simulink model "TeamA_PAsqualo1"  (R2020a)
settings: Solver=VariableStepAuto  StartTime=0.0  StopTime=stop_time  FixedStep=0.05  RelTol=1e-3
InitFcn:
  | main_init
values from neighbouring files (symbols this model uses):
  a1 = rho * D^4 * alpha1    (= 0.000388302366464)    [data_current.m]    (also in main_init.m)
  a2 = -rho * D^3 * alpha2 * (1 - omega)    (= 0.0037030698432)    [data_current.m]    (also in main_init.m)
  ag = [Ax Ay Az]'    [init_modello.m]
  alpha1 = 0.0113    [data_current.m]    (also in main_init.m)
  alpha2 = -0.0091    [data_current.m]    (also in main_init.m)
  areaOfInterestCorner = [42.317744;10.915136; 0]    [init_controllo.m]    (also in missionA.m = [42.317744)
  bg = [Bx By Bz]'    [init_modello.m]
  cd_pitch = 0.7    [init_modello.m]
  cd_roll = 0.04    [init_modello.m]
  cd_x = 0.4    [init_modello.m]
  cd_y = 1    [init_modello.m]
  cd_yaw = 0.7    [init_modello.m]
  cd_z = 1    [init_modello.m]
  cg = [Cx Cy Cz]'    [init_modello.m]
  D = 0.076    [data_current.m]    (also in main_init.m)
  dead_zone_limit = 31.5    [data_current.m]    (also in main_init.m)
  dg = [Dx Dy Dz]'    [init_modello.m]
  eg = [Ex Ey Ez]'    [init_modello.m]
  fg = [Fx Fy Fz]'    [init_modello.m]
  g = 9.81    [init_modello.m]
  galleggiamento = 66.5386    [init_controllo.m]
  gg = [Gx Gy Gz]'    [init_modello.m]
  H0 = 0    [init_modello.m]
  init_position = [pointP(1),pointP(2),0.15,0,0,deg2rad(angle)]'    [appunti.m]    (also in init_modello.m = [pointP(1),pointP(2),0.15,0,0,deg2rad(alpha)]')
  init_velocity = [0 0 0 0 0 0]'    [init_modello.m]
  initial_state_cov = blkdiag(diag(cov_gps(1,1:2)), cov_depth*eye(n_state_filter-2))    [init_navigazione.m]
  Ixx = 0.93304097392    [init_modello.m]
  Ixy = 0    [init_modello.m]
  Ixz = 0    [init_modello.m]
  Iyy = 25.58745481378    (= 25.5874548138)    [init_modello.m]
  Iyz = 0    [init_modello.m]
  Izz = 25.58745481378    (= 25.5874548138)    [init_modello.m]
  K_i_heave_div = 20    [init_controllo.m]
  K_i_heave_pos = 1    [init_controllo.m]
  K_i_heave_surf = 20    [init_controllo.m]
  K_i_heave_trans = 5    [init_controllo.m]
  K_i_heave_turn = 5    [init_controllo.m]
  K_i_pitch_div = 0    [init_controllo.m]
  K_i_pitch_pos = 0.1*0    (= 0)    [init_controllo.m]
  K_i_pitch_surf = 0    [init_controllo.m]
  K_i_pitch_trans = 0    [init_controllo.m]
  K_i_pitch_turn = 0    [init_controllo.m]
  K_i_roll_div = 0    [init_controllo.m]
  K_i_roll_pos = 0.1*0    (= 0)    [init_controllo.m]
  K_i_roll_surf = 1    [init_controllo.m]
  K_i_roll_trans = 0    [init_controllo.m]
  K_i_roll_turn = 0    [init_controllo.m]
  K_i_surge_div = 3    [init_controllo.m]
  K_i_surge_pos = 0.1679*30    (= 5.037)    [init_controllo.m]
  K_i_surge_surf = 3    [init_controllo.m]
  K_i_surge_trans = 0.1679*15    (= 2.5185)    [init_controllo.m]
  K_i_surge_turn = 0.1679*60    (= 10.074)    [init_controllo.m]
  K_i_sway_div = 6    [init_controllo.m]
  K_i_sway_pos = 5    [init_controllo.m]
  K_i_sway_surf = 3    [init_controllo.m]
  K_i_sway_trans = 2    [init_controllo.m]
  K_i_sway_turn = 50    [init_controllo.m]
  K_i_yaw_div = 0    [init_controllo.m]
  K_i_yaw_pos = 1    [init_controllo.m]
  K_i_yaw_surf = 0    [init_controllo.m]
  K_i_yaw_trans = 20    [init_controllo.m]
  K_i_yaw_turn = 3    [init_controllo.m]
  K_p_heave_div = 200    [init_controllo.m]
  K_p_heave_pos = 320    [init_controllo.m]
  K_p_heave_surf = 200    [init_controllo.m]
  K_p_heave_trans = 170    [init_controllo.m]
  K_p_heave_turn = 170    [init_controllo.m]
  K_p_phi_div = 0.15    [init_controllo.m]
  K_p_phi_pos = 1*0.1    (= 0.1)    [init_controllo.m]
  K_p_phi_surf = 0.15    [init_controllo.m]
  K_p_phi_trans = 0.1    [init_controllo.m]
  K_p_phi_turn = 0.1    [init_controllo.m]
  K_p_pitch_div = 50    [init_controllo.m]
  K_p_pitch_pos = 25    [init_controllo.m]
  K_p_pitch_surf = 50    [init_controllo.m]
  K_p_pitch_trans = 25    [init_controllo.m]
  K_p_pitch_turn = 25    [init_controllo.m]
  K_p_psi_div = 0.3    [init_controllo.m]
  K_p_psi_pos = 0.25    [init_controllo.m]
  K_p_psi_surf = 0.3    [init_controllo.m]
  K_p_psi_trans = 0.2    [init_controllo.m]
  K_p_roll_div = 10    [init_controllo.m]
  K_p_roll_pos = 0.1*40    (= 4)    [init_controllo.m]
  K_p_roll_surf = 10    [init_controllo.m]
  K_p_roll_trans = 0.1*40    (= 4)    [init_controllo.m]
  K_p_roll_turn = 4    [init_controllo.m]
  K_p_surge_div = 80    [init_controllo.m]
  K_p_surge_pos = 13.7782*2.5    (= 34.4455)    [init_controllo.m]
  K_p_surge_surf = 80    [init_controllo.m]
  K_p_surge_trans = 20    [init_controllo.m]
  K_p_surge_turn = 150    [init_controllo.m]
  K_p_sway_div = 100    [init_controllo.m]
  K_p_sway_pos = 90    [init_controllo.m]
  K_p_sway_surf = 80    [init_controllo.m]
  K_p_sway_trans = 80    [init_controllo.m]
  K_p_sway_turn = 200    [init_controllo.m]
  K_p_th_div = 0.3    [init_controllo.m]
  K_p_th_pos = 0.1    [init_controllo.m]
  K_p_th_surf = 0.3    [init_controllo.m]
  K_p_th_trans = 0.1    [init_controllo.m]
  K_p_th_turn = 0.1    [init_controllo.m]
  K_p_x_div = 0.12    [init_controllo.m]
  K_p_x_pos = 0.12    [init_controllo.m]
  K_p_x_surf = 0.12    [init_controllo.m]
  K_p_y_div = 0.6    [init_controllo.m]
  K_p_y_pos = 0.34    [init_controllo.m]
  K_p_y_surf = 0.1    [init_controllo.m]
  K_p_y_trans = 0.3    [init_controllo.m]
  K_p_y_turn = 0.3    [init_controllo.m]
  K_p_yaw_div = 70    [init_controllo.m]
  K_p_yaw_pos = 20    [init_controllo.m]
  K_p_yaw_surf = 70    [init_controllo.m]
  K_p_yaw_trans = 160    [init_controllo.m]
  K_p_yaw_turn = 60    [init_controllo.m]
  K_p_z_div = 0.35    [init_controllo.m]
  K_p_z_pos = 0.2    [init_controllo.m]
  K_p_z_surf = 0.35    [init_controllo.m]
  K_p_z_trans = 0.10    (= 0.1)    [init_controllo.m]
  K_p_z_turn = 0.1    [init_controllo.m]
  Kadd = 0    [init_modello.m]
  ... (+61 more)
undefined symbols (not defined in the file or in its folder): DiscIntNeverNeededParam, initial_state
libraries: simulink x4, vrlib x1
(part 4 of 6)

== matlab function TeamA_PAsqualo1/Navigazione/Predizione/predizione_propagate ==
  data: mean input size=[n_state_aug_filter 1]; mean_new output size=[n_state_filter, 1]; cov input size=[n_state_aug_filter n_state_aug_filter]; cov_new output size=[n_state_filter n_state_filter]; n_state_aug_filter parameter; ts_filter parameter; n_state_filter parameter
function [mean_new, cov_new] = propagate(mean, cov, n_state_aug_filter, ts_filter, n_state_filter)
 % PROPAGATE genera un numero n di sigma points, li propaga attraverso
 % state_update e da` come output la media e la covarianza dei nuovi sigma
 % points. 
 %
 % Input		
 % mean			vettore media dello stato nx1
 % cov			matrice covarianza dello stato nxn
 %
 % Output
 % mean_new		vettore media dello stato nx1
 % cov_new		matrice covarianza dello stato nxn

[sp, wm, wc] = sigmapoint_gen(mean, cov, n_state_aug_filter);

[mean_new, P] = sigmapoint_propagate(sp, wm, wc, ...
					n_state_aug_filter, ts_filter, n_state_filter);

% check simmetria
cov_new = (P + P')/2;

end

%--------------------------------------------------------------------------
%--------------------------------------------------------------------------
function state_new = state_update(state_aug, ts_filter)


pos = state_aug(1:3, 1);
ahrs = state_aug(4:6, 1); % roll pitch yaw
dvl = state_aug(7:9, 1);

% yaw, pitch, roll
Rbn = rotz(ahrs(3))' * roty(ahrs(2))' * rotx(ahrs(1))';

state_new = pos + ts_filter * Rbn * dvl;

end

function Rx = rotx(ang)

Rx = [	1 0 0; ...
		0 cos(ang) sin(ang); ...
		0 -sin(ang) cos(ang)];

end
function Ry = roty(ang)

Ry = [	cos(ang) 0 -sin(ang); ...
		0 1 0; ...
		sin(ang) 0 cos(ang)];

end
function Rz = rotz(ang)

Rz = [	cos(ang) sin(ang) 0; ...
		-sin(ang) cos(ang) 0; ...
		0	0 1];

end
		
%--------------------------------------------------------------------------
%--------------------------------------------------------------------------
function [sp, wm, wc] = sigmapoint_gen(mean, cov, n_state_filter)
% questa funzione genera i sigma point e i loro pesi
	

	n		= n_state_filter;	% Dimensione dello spazio in cui vengono generati
	nsp		= 2*n+1;			% numero di sigma points. in generale pari a (2n+1)
	P       = cov;				% matrice di covarianza
%	mean    = mean;				%
	
	% par da rivedere
	alpha	= 1;
	beta	= 2;
	k		= 0;
    
	%   
	lambda = alpha^2 * (n + k) -n;
	
	% generazione pesi per media
	wm = 1/(2*(n + lambda)) * ones(nsp, 1);
    wm(1) = lambda/(n + lambda);
	
	% generazione pesi per cov
	wc = 1/(2*(n + lambda)) * ones(nsp, 1);
	wc(1) = lambda/(n + lambda) + (1 - alpha^2 + beta);
	
	% generazione sigma points sp
	dist = zeros(n_state_filter,n_state_filter);
	sp = zeros(n_state_filter, nsp);
	
	[U, SIGMA, ~] = svd((n+lambda)* P);
	dist = U * sqrt(SIGMA);

	for i=1:nsp
		if i == 1
			sp(:,i) = mean;
		elseif i<=1+n
			sp(:,i) = mean+dist(:,i-1);
		elseif i>1+n && i<=nsp
			sp(:,i) = mean-dist(:,i-1-n);
		end
	end

end

%--------------------------------------------------------------------------
%--------------------------------------------------------------------------
function [mean_new, cov_new] = sigmapoint_propagate(sp, wm, wc, n_state_aug_filter, ts_filter, n_state_filter)
% questa funzione propaga i sigma point usando state_update
	
	
	nsp = n_state_aug_filter*2 + 1;
	sp_new = zeros(n_state_filter, nsp);
	for j = 1:nsp
		 sp_new(:,j) = state_update(sp(:,j), ts_filter);
	end

	% media
	mean_new = zeros(n_state_filter, 1);
	for j = 1:nsp
		mean_new = mean_new + wm(j)*sp_new(:,j);
	end

	% cov
	cov_new = zeros(n_state_filter, n_state_filter);  
	for j = 1:nsp
		 cov_new = cov_new + wc(j)*(sp_new(:,j) - mean_new)*(sp_new(:,j) - mean_new)';
	end

	
end

== matlab function TeamA_PAsqualo1/Navigazione/Predizione/smart_mux ==
  data: x_mean input size=[n_state_filter 1]; mean output size=[9 1]; x_cov input size=[n_state_filter n_state_filter]; u_mean input size=[n_input_filter 1]; u_cov input size=[n_input_filter n_input_filter]; cov output size=[n_state_aug_filter, n_state_aug_filter]; n_state_filter parameter; n_input_filter parameter
function [mean, cov] = smart_mux(x_mean, x_cov, u_mean, u_cov, n_state_filter, n_input_filter)

% init
mean = zeros(n_state_filter+n_input_filter, 1);
mean = [x_mean; u_mean];
    
cov = zeros(n_state_filter + n_input_filter);
cov = blkdiag(x_cov, u_cov);

end

== matlab function TeamA_PAsqualo1/Navigazione/Predizione Misure/propagazione misura NED1 ==
  data: x input; P input; y_virt output size=[5 1]; S_virt output; C output; n_state_filter parameter; n_meas_filter parameter; pos_transp parameter; p_usbl parameter; or input
function [y_virt, S_virt, C] = propagazione_misure(x, P, n_state_filter, n_meas_filter, pos_transp, p_usbl, or)
 % PROPAGATE_MISURE genera i sigma points, li propaga attraverso state2meas
 % e da` come output la media, la covarianza dei nuovi sigma points e la 
 % crosscovarianza stato-meas.
 %
 % Input		
 % mean			vettore media dello stato nx1
 % cov			matrice covarianza dello stato nxn
 %
 % Output
 % mean_new		vettore media dello misure mx1
 % cov_new		matrice covarianza dello delle misure mxm
 % C			matrice crosscovarianza nxm


[sp, wm, wc] = sigmapoint_gen(x, P, n_state_filter);

[~, y_virt, esse, C] = sigmapoint_propagate(sp, x, wm, wc, n_state_filter, ...
									n_meas_filter, pos_transp, p_usbl, or);

% check simmetria								
S_virt = (esse + esse')/2;


end

%--------------------------------------------------------------------------
%--------------------------------------------------------------------------
function meas = state2meas(state, n_meas_filter, pos_transp,  p_usbl, or)

meas = zeros(n_meas_filter,1);

Rbn = rotz(or(3))' * roty(or(2))' * rotx(or(1))';

% ned2usbl
pos_sensore_onboard = state(1:3,1) + Rbn*p_usbl;

vettore_auv_trasp =  +(pos_transp - pos_sensore_onboard) ;
range	= norm(vettore_auv_trasp,2);
bear	= atan2(vettore_auv_trasp(2),vettore_auv_trasp(1));

% depth
meas_depth = state(3);


meas = [state(1); state(2); bear; range; meas_depth];

end


function Rx = rotx(ang)

Rx = [	1 0 0; ...
		0 cos(ang) sin(ang); ...
		0 -sin(ang) cos(ang)];

end
function Ry = roty(ang)

Ry = [	cos(ang) 0 -sin(ang); ...
		0 1 0; ...
		sin(ang) 0 cos(ang)];

end
function Rz = rotz(ang)

Rz = [	cos(ang) sin(ang) 0; ...
		-sin(ang) cos(ang) 0; ...
		0	0 1];

end

%--------------------------------------------------------------------------
%--------------------------------------------------------------------------
function [sp, wm, wc] = sigmapoint_gen(mean, cov, n_state_filter)
% questa funzione genera i sigma point e i loro pesi


	n		= n_state_filter;	% Dimensione dello spazio in cui vengono generati
	nsp		= 2*n+1;			% numero di sigma points. in generale pari a (2n+1)
	P       = cov;				% matrice di covarianza
%	mean    = mean;				%
	
	% par da rivedere
	alpha	= 1;
	beta	= 2;
	k		= 0;
    
	%   
	lambda = alpha^2 * (n + k) -n;
	
	% generazione pesi per media
	wm = 1/(2*(n + lambda)) * ones(nsp, 1);
    wm(1) = lambda/(n + lambda);
	
	% generazione pesi per cov
	wc = 1/(2*(n + lambda)) * ones(nsp, 1);
	wc(1) = lambda/(n + lambda) + (1 - alpha^2 + beta);
	
	% generazione sigma points sp
	[U, SIGMA, ~] = svd((n+lambda)* P);
	dist = U * sqrt(SIGMA);
	
	sp = zeros(n_state_filter, nsp);
	for i=1:nsp
		if i == 1
			sp(:,i) = mean;
		elseif i<=1+n
			sp(:,i) = mean+dist(:,i-1);
		elseif i>1+n && i<=nsp
			sp(:,i) = mean-dist(:,i-1-n);
		end
	end
	%sp = [mean mean+dist(:,1) mean+dist(:,2) mean-dist(:,1) mean-dist(:,2)];
	%sp = [mean mean+dist mean-dist];

end

%--------------------------------------------------------------------------
%--------------------------------------------------------------------------
function [sp_new, mean_new, cov_new, C] = sigmapoint_propagate(sp, mean, wm, wc, n_state_filter, n_meas_filter, pos_transp, p_usbl, or)
% questa funzione propaga i sigma point usando state_update

	nsp = n_state_filter*2 + 1;
	
	sp_new = zeros(n_meas_filter, nsp);
	
	for j = 1:nsp
		%	state2meas(state, n_state_filter, n_meas_filter, ned_origin, spheroid)
		sp_new(:,j) = state2meas(sp(:,j), n_meas_filter,...
						pos_transp, p_usbl, or);
	end

	% media
	mean_new = mean_func(n_meas_filter, sp_new, wm, nsp);

	% cov
	[cov_new, C] = cov_func(sp, mean, sp_new, mean_new, wc, nsp, n_meas_filter, n_state_filter);
	
end

%--------------------------------------------------------------------------
%--------------------------------------------------------------------------
function mean_new = mean_func(n_meas_filter, sp_new, wm, nsp)
% ymeas = 	lat
% 			lon
% 			bear
% 			range
% 			depth

mean_new = zeros(n_meas_filter, 1);

for j = 1:nsp
	mean_new = mean_new + wm(j)*sp_new(:,j);
end

%calcolo media bearing :)
mean_c = 0;
mean_s = 0;
for j = 1:nsp
	c = cos(sp_new(3,j));
	s = sin(sp_new(3,j));
	
	mean_c = mean_c + wm(j)*c;
	mean_s = mean_s + wm(j)*s;
end
mean_new(3) = atan2(mean_s, mean_c);

end

%--------------------------------------------------------------------------
%--------------------------------------------------------------------------
function [cov_new, C] = cov_func(sp, mean, sp_new, mean_new, wc, nsp, n_meas_filter, n_state_filter)
% ymeas = 	lat
% 			lon
% 			bear
% 			range
% 			depth

% init
cov_new = zeros(n_meas_filter, n_meas_filter);  

C = zeros(n_state_filter, n_meas_filter);


% covarianza uscite non angolari
b = zeros(n_meas_filter, 1);
for j = 1:nsp
    b = sp_new(:,j) - mean_new(:,1);
    cov_new = cov_new + wc(j) * (b*b');
end

%covarianza bearing
cc = 0;
cs = 0;
for j = 1:nsp
	c = cos(sp_new(3,j) - mean_new(3));
	s = sin(sp_new(3,j) - mean_new(3));
	
	cc = cc + wc(j)*(c*c');
	cs = cs + wc(j)*(s*s');
end
cov_new(3,3) = atan2(cs,cc);


%----------------------------------------------------
% Calcolo Crosscovarianza
% 
% [	x1y1 x1y2 x1y3 x1y4 x1y5;
% 	x2y1 x2y2 x2y3 x2y4 x2y5;
% 	x3y1 x3y2 x3y3 x3y4 x3y5 
%	x4y1 x4y2 x4y3 x4y4 x4y5]

C = zeros(n_state_filter, n_meas_filter);
for j = 1:nsp
	
	C = C + wc(j)*((sp(:,j)-mean)*(sp_new(:,j) ...
								- mean_new(:,1))');
end

%covarianza bearing 
Cb = zeros(n_state_filter,1);
for j = 1:nsp
	ang = sp_new(3,j)- mean_new(3,1);
	a = atan2(sin(ang),cos(ang));
	Cb = Cb + wc(j)*((sp(:,j)-mean)*a);
end
C(:,3) = Cb;
end

== matlab function TeamA_PAsqualo1/Navigazione/Selettore Misure/Selettore misure/MATLAB Function ==
  settings: updateMethod=DISCRETE
  data: col output size=[1 5]; u input; row output size=[1 5]; run output
function [col ,row, run] = select(u)

    run = 0;
    row = [];
    col = [];
    
    if u(1) == 1 % gps
        row = [row 1 2];
        col = [col 1 2];
        run = 1;
    end
    if u(2) == 1 % usbl
        row = [row 3 4];
        col = [col 3 4];
        run = 1;
    end
    if u(3) == 1 % depth
        row = [row 5];
        col = [col 5];
        run = 1;
    end

   
end

== matlab function TeamA_PAsqualo1/Navigazione/Selettore Misure/Selettore misure/pulse/MATLAB Function ==
  data: gps_now input size=[2,1]; u input; y output; ned_origin parameter
function y  = tolo_pulse(gps_now,u, ned_origin)
% questa funzione fornisce 1 se il valore in ingresso e` cambiato rispetto al
% time step precendente, 0 altrienti
coder.extrinsic('evalin', 'wgs84Ellipsoid', 'geodetic2ned');
nogps_lat = 0;
nogps_lon = 0;
[nogps_lat, nogps_lon, ~] = geodetic2ned(...
											0, 0, 0,...
											ned_origin(1), ned_origin(2), ned_origin(3),...
											wgs84Ellipsoid);


if (gps_now(1)==nogps_lat && gps_now(2)==nogps_lon)
	%gps non funzionante
	y = 0;
elseif norm(u) == 0
    y = 0;
else
    y = 1;
end



end

== matlab function TeamA_PAsqualo1/Navigazione/Selettore Misure/Selettore misure/pulse2/MATLAB Function ==
  data: u input; y output
function y  = tolo_pulse(u)
% questa funzione fornisce 1 se il valore in ingresso e` cambiato rispetto al
% time step precendente, 0 altrienti

if norm(u) == 0
    y = 0;
else
    y = 1;
end

end

== matlab function TeamA_PAsqualo1/Navigazione/Selettore Misure/Selettore misure/pulse4/MATLAB Function ==
  data: u input; y output
function y  = tolo_pulse(u)
% questa funzione fornisce 1 se il valore in ingresso e` cambiato rispetto al
% time step precendente, 0 altrienti

if norm(u) == 0
    y = 0;
else
    y = 1;
end

end

== matlab function TeamA_PAsqualo1/Navigazione/dvl2body ==
  data: ni_dvl input; ni output; omega input; p_dvl parameter
function ni = fondcine(ni_dvl, omega, p_dvl)

% dist_dvl_body e` il vettore che va dall'origine del sistema di riferimento 
% body al sensore dvl
 
ni = ni_dvl + cross(omega, -p_dvl);


end

== matlab function TeamA_PAsqualo1/Navigazione/geo2ned1 ==
  data: geo input; ned output size=[3 1]; ned_origin parameter
function ned = geo2ned(geo, ned_origin)
coder.extrinsic('evalin', 'wgs84Ellipsoid', 'geodetic2ned');

[x, y, z] = geodetic2ned(geo(1), geo(2), geo(3),ned_origin(1), ned_origin(2), ned_origin(3), wgs84Ellipsoid);

ned = zeros(3,1);
ned = [x;y;z];
end

== matlab function TeamA_PAsqualo1/Navigazione/geo2ned2 ==
  data: ned input; LLD output size=[3 1]; ned_origin parameter
function LLD = ned2lld(ned, ned_origin)
coder.extrinsic('evalin', 'wgs84Ellipsoid', 'ned2geodetic');

[Lat, Lon, z] = ned2geodetic(ned(1), ned(2), 0,ned_origin(1), ned_origin(2), ned_origin(3), wgs84Ellipsoid);

LLD = zeros(3,1);
LLD = [Lat; Lon; ned(3)];
end

== stateflow chart TeamA_PAsqualo1/Mission Supervisor2/Chart ==

== stateflow chart TeamA_PAsqualo1/Mission Supervisor2/State Management ==
  state Movements [parallel]
    settings: executionOrder=1
    state End [function]
    state positioning
      entry:
      current_state(1:5) = [1 0 0 0 0];
      orBene = 0;
      velNull = 0;
      fromFirstPos = 0;
      during:
      if ~missionEnd %missione appena iniziata
      if ~checkOr([0,0,orDes],orient,errOrPos) && ~orBene
      pos_ref = pointP;
      orient_ref = [0,0,orDes];
      vel_ref = [0,0,0,0,0,0];
      else%orientato bene, dentro o fuori sfera
      orBene=1;
      pos_ref = pointA;
      orient_ref = [0,0,orDes];
      vel_ref = velPos;
      end
      else %missione completata con successo
      pos_ref = pointP;
      orient_ref = [0,0, orDesRit];
      vel_ref = velPos;
      end
    state diving
      entry:
      current_state(1:5) = [0 1 0 0 0];
      velNull = 0;
      during:
      if ~(checkPos(pointA,pos, errSphere) && checkOr([0,0,orDes],orient,errOrPos) ...
      && checkVel(zeros(1,6),[vel(1),vel(2),vel(3),0,0,0],errVelDiv)) && ~velNull
      pos_ref = pointA;
      orient_ref = [0,0,orDes];
      vel_ref = zeros(1,6);
      else
      velNull = 1;
      pos_ref = [pointA(1),pointA(2), averageDepth - altitude];
      orient_ref = orientA;
      if (pos_ref(3) - pos(3) > endDiv)
      vel_ref = velSub;
      else
      vel_ref = velRidSub;
      end
      end
    state surfacing
      entry:
      current_state(1:5) = [0 0 0 0 1];
      velNull = 0;
      during:
      if wall || current_state(8)
      pos_ref = [pos(1), pos(2), 0.15];
      vel_ref = [0 0 0.2 0 0 0];
      else
      if ~checkVel(zeros(1,6),[vel(1),vel(2),vel(3),0,0,0],errVelSurf) && ~velNull
      pos_ref = trWP(nWPTran,:,nTran);
      orient_ref = [0,0,orDesRit];
      vel_ref = zeros(1,6);
      else
      velNull = 1;
      ptSup = trWP(nWPTran,:,nTran);
      pos_ref = [ptSup(1),ptSup(2),0.15];
      orient_ref = [0,0,orDesRit];
      vel_ref = velSurf;
      end
      end
    state transect
      entry:
      current_state(1:5) = [0 0 1 0 0];
      ptx = trWP(wpTR,:,page);
      pos_ref = [ptx(1),ptx(2),pos(3)-(altitude-FLS_down)];
      if mod(page,2) == 0
      orient_ref = orPari;
      else
      orient_ref = orDispari;
      end
      vel_ref = velTran;
      state Disaligned
        (default) -> (junction 490)
        (junction 490) -> (junction 207) : {sizeEmerg = size(wpEmerg);}
        (junction 207) -> (junction 674) [order 1] : [~all(sizeEmerg)]
        (junction 674) -> (junction 681) [order 2] : {wpTR = nWPTran;}
        (junction 207) -> (junction 210) [order 2]
        (junction 674) -> (junction 681) [order 1] : [wpTR + 2 <= nWPTran]
            | {wpTR = wpTR+2;}
        (junction 681) -> (junction 210) : {wpEmerg = currentSwingWaypoints(trWP(wpTR,:,page),pos,distEmerg);}
        (junction 210) -> (junction 396) : {ptx = wpEmerg(idxEmerg,1:3);
            | pos_ref = [ptx(1),ptx(2),pos(3)-(altitude-FLS_down)];
            | vel_ref = vEmergTran;}
        (junction 396) -> (junction 225) [order 1] : [mod(page,2) == 0]
            | {orient_ref = orPari;}
        (junction 396) -> (junction 225) [order 2] : {orient_ref =orDispari;}
        (junction 225) -> (junction 259) [order 2]
        (junction 225) -> (junction 213) [order 1] : [checkPos(pos,pos_ref,errPosWPTrans) &&...
            | checkOr(orient,orient_ref,errOrWPTrans)]
        (junction 213) -> (junction 215) [order 1] : [idxEmerg == size(wpEmerg,1)]
            | {idxEmerg = 1; current_state(6) = 0;}
        (junction 213) -> (junction 215) [order 2] : {idxEmerg = idxEmerg + 1;}
      state Aligned
        (default) -> (junction 203)
        (junction 203) -> (junction 754) [order 2] : {error=errPosTransLast;}
        (junction 203) -> (junction 754) [order 1] : [wpTR<=nWPTran-2]
            | {error=errPosTrans;}
        (junction 754) -> (junction 219) [order 2]
        (junction 754) -> (junction 663) [order 1] : [checkPos(pos_ref,pos,error) && ...
            | checkOr(orient_ref,orient,errOrTrans)]
        (junction 663) -> (junction 219) : [wpTR+1 <= nWPTran]
            | {wpTR = wpTR + 1;} %indica WP successivo
        (junction 219) -> (junction 393) : {wpEmerg =  [];
            | ptx = trWP(wpTR,:,page);
            | pos_ref = [ptx(1),ptx(2),pos(3)-(altitude-FLS_down)];}
        (junction 393) -> (junction 222) [order 1] : [mod(page,2) == 0]
            | {orient_ref = orPari;}
        (junction 393) -> (junction 222) [order 2] : {orient_ref = orDispari;}
        (junction 222) -> (junction 227) [order 1] : [wpTR > nWPTran - 2]
            | {vel_ref = velRid;}
        (junction 222) -> (junction 227) [order 2] : {vel_ref = velTran;}
      Aligned -> Aligned [order 2]
      Disaligned -> Disaligned [order 2]
      (default) -> Aligned
      Disaligned -> Aligned [order 1] : [~current_state(6)]
      Aligned -> Disaligned [order 1] : [current_state(6)]
    state turn
      entry:
      current_state(1:5) = [0 0 0 1 0];
      state ReferencePoints
        (default) -> (junction 728)
        (junction 728) -> (junction 736) [order 2] : {pos_ref = turnWP(nWPTurn,:,page);
            | orient_ref = deg2rad(turnRef(nWPTurn,:,page));}
        (junction 728) -> (junction 733) [order 1] : [time+1<=nWPTurn]
            | {pos_ref = turnWP(time+1,:,page);
            | orient_ref = deg2rad(turnRef(time+1,:,page));}
        (junction 736) -> (junction 733)
        (junction 733) -> (junction 738) [order 1] : [mod(page,2) == 0]
            | {vel_ref = [0.2 0 0 0 0 -rot*0.2/(lineSpaceBetweenTransects/2)];}
        (junction 733) -> (junction 731) [order 2] : {vel_ref = [0.2 0 0 0 0 rot*0.2/(lineSpaceBetweenTransects/2)];}
      ReferencePoints -> ReferencePoints
      (default) -> ReferencePoints
    (default) -> positioning : {missionEnd = 0;}
    positioning -> positioning [order 1] : [missionEnd && checkPos(pointP,pos,errPosPos/2)]
        | {End();}
    positioning -> diving [order 2] : [checkPos(pointA,pos,errPosPos) && checkOr([0,0,orDes],orient,errOrPos)]
    positioning -> surfacing [order 3] : [wall || current_state(8)]
        | {fromFirstPos = 1;}
    surfacing -> positioning : [checkPos3([ptSup(1),ptSup(2),0.15],pos,errPosSurf) && ...
        | checkOr([0,0,orDesRit],orient,errOrSurf) && checkVel(zeros(1,6),vel,errVelSurf)...
        | && ~fromFirstPos]
        | {missionEnd = 1;}
    diving -> surfacing [order 2] : [wall || current_state(8)]
    diving -> transect [order 1] : [checkPos3([pointA(1),pointA(2), pos(3)-(altitude-FLS_down)],pos,errPosDiv) ...
        | && checkOr(orientA,orient,errOrDiv)]
    transect -> surfacing [order 1] : [wall || current_state(8)]
    turn -> surfacing [order 2] : [wall || current_state(8)]
    transect -> surfacing [order 2] : [(checkPos(trWP(nWPTran,:,nTran),pos, errPosTrans) &&...
        | checkOr(orient_ref,orient,errOrTrans))]
    (junction 830) -> transect [order 2] : {wpTR = 1;}
    turn -> (junction 830) [order 1] : [time+1 == nWPTurn]
        | {page = page + 1;}
    (junction 830) -> transect [order 1] : [cruiseSpeed>=1.5 && lineSpaceBetweenTransects<4]
        | {wpTR = 2;}
    transect -> turn [order 3] : [checkPos(trWP(nWPTran,:,page),pos, errPosTransLast) && checkOr(orient_ref,orient,errOrTrans)]
        | {wpTU=1;}
  state Issues_management [parallel]
    entry:
    points=[];
    profs=[];
    settings: executionOrder=2
    state Free
      entry:
      current_state(6:8) = 0;
      during:
      if current_state(1) || current_state(5)
      pos_ref(3) = 0.15;
      else
      if abs(altitude - FLS_down)>=minGap
      pos_ref(3)= pos(3) - (altitude - FLS_down);
      else
      pos_ref(3) = pos(3);
      end
      end
    state Issue_found
      state obstacle %parete/ostacoli [parallel]
        entry,during:
        distFront = FLS_front*cos(deg2rad(theta_f));
        distDown = FLS_front*sin(deg2rad(theta_f));
        oDeg= rad2deg(orient);
        nedFLS = fix2LocalNED(oDeg(1),oDeg(2),oDeg(3))'*[distFront;0;distDown];
        pointProf = pos(3) - (altitude-FLS_down) - (FLS_down-nedFLS(3));
        pointApp = calcPoint(pos,oDeg,nedFLS(1));
        nedAxis = (fix2LocalNED(oDeg(1),oDeg(2),oDeg(3))'*[semix; semiy; semiz])';
        settings: executionOrder=3
        (default) -> (junction 563)
        (junction 563) -> (junction 800) [order 1] : [~current_state(3)]
            | {points = [];profs=[];}
        (junction 563) -> (junction 575) [order 3] : [~all(size(points))]
            | %{current_state(7) = 0;}
        (junction 563) -> (junction 565) [order 2] : [all(size(points))]
            | {distObsVeh = distance(pos+nedAxis,points(1,:));
            | punto = points(1,:);}
        (junction 565) -> (junction 789) [order 2] : [distObsVeh>(abs(pos(3)-profs(1))...
            | /maxRatio + safeMargin)]
        (junction 565) -> (junction 567) [order 1] : [distObsVeh<=(abs(pos(3)-profs(1))/maxRatio + safeMargin)]
            | {pos_ref(3) = profs(1);}
        (junction 575) -> (junction 573)
        (junction 567) -> (junction 791)
        (junction 789) -> (junction 791)
        (junction 791) -> (junction 573) [order 2]
        (junction 791) -> (junction 573) [order 1] : [checkPos([punto(1),punto(2),profs(1)],pos,errPosPos)]
            | {points  = points(2:end,:);}
        (junction 573) -> (junction 578) [order 1] : [abs(pos(3) - pointProf)/(distFront+nedAxis(1)) > maxRatio]
            | {current_state(7) = 1;wall = 1;}
        (junction 573) -> (junction 605) [order 3]
        (junction 573) -> (junction 580) [order 2] : [abs(pos(3) - pointProf)/(distFront+nedAxis(1)) <= maxRatio]
        (junction 580) -> (junction 582) [order 1] : [all(size(points))]
            | {distObs = distance(points(end,:),pointApp);}
        (junction 580) -> (junction 794) [order 2] : [~all(size(points))]
        (junction 794) -> (junction 796) [order 2]
        (junction 794) -> (junction 586) [order 1] : [abs(pos(3)-pointProf)>=minGap]
            | {distObsVeh=distance(pos,pointApp);}
        (junction 582) -> (junction 785) [order 2]
        (junction 582) -> (junction 584) [order 1] : [abs(profs(end)-pointProf)>=minGap]
        (junction 586) -> (junction 787) [order 2]
        (junction 586) -> (junction 588) [order 1] : [distObsVeh>=minDist+nedAxis(1)]
            | {points = addP(points,pointApp);}
            | %cat(1,points,pointApp);}
        (junction 584) -> (junction 590) [order 1] : [distObs < minDist || abs(profs(end)-pointProf)/distObs > maxRatio]
            | {points = points(1:end-1,:);}
        (junction 584) -> (junction 592) [order 2]
        (junction 590) -> (junction 592)
        (junction 592) -> (junction 595) : {points=addP(points,pointApp);}
            | %cat(1,points,pointApp);}
      state warning %disallineamento [parallel]
        during:
        if current_state(3)
        disalignOP;
        end
        if current_state(1) || current_state(5)
        pos_ref(3) = 0.15;
        else
        if abs(altitude - FLS_down)>=minGap
        pos_ref(3)= pos(3) - (altitude - FLS_down);
        else
        pos_ref(3) = pos(3);
        end
        end
        settings: executionOrder=1
      state abort %danni strutturali [parallel]
        entry:
        inactivity = 1;
        during:
        checkFailure;
        settings: executionOrder=2
      state disalignOP [function]
        (default) -> (junction 696)
        (junction 696) -> (junction 700) [order 1] : [current_state(3) && wpTR >=2 &&...
            | retta(pos,trWP(1,:,page),trWP(nWPTran,:,page))>=offset]
            | {current_state(6) = 1;}
        (junction 696) -> (junction 747) [order 2] : [current_state(3) && wpTR>nWPTran-2 ...
            | && retta(pos,trWP(1,:,page),trWP(nWPTran,:,page))>=offsetLast]
            | {current_state(6) = 1;}
        (junction 696) -> (junction 780) [order 3]
      state checkFailure [function]
        (default) -> (junction 108)
        (junction 109) -> (junction 114) : [mod(inactivity,1000) == 0]
            | {current_state(8) = 1;}
        (junction 108) -> (junction 109) : [vel(1:3) == [0 0 0]]
            | {inactivity = inactivity + 1;}
    state rit = check [function]
      (default) -> (junction 122)
      (junction 122) -> (junction 479) [order 2] : {rit = 0;}
      (junction 122) -> (junction 124) [order 1] : [(current_state(3) && wpTR >=2 &&...
          | retta(pos,trWP(1,:,page),trWP(nWPTran,:,page))>=offset) ||...
          | current_state(3) && wpTR>nWPTran-2 ...
          | && retta(pos,trWP(1,:,page),trWP(nWPTran,:,page))>=offsetLast ||...
          |  all(size(points)) ]
          | {rit = 1;}
    (default) -> Free
    Free -> Issue_found : [check]
    Issue_found -> Free : [~check]
  data: puntoDes function_input; puntoCorr function_input; dist function_input; M function_output; ang constant double =angle; vRef function_input; vAct function_input; vErr function_input; okVel function_output; oRef function_input; oAct function_input; oErr function_input; okOr function_output; pRef function_input; pAct function_input; pErr function_input; okPos function_output; pRef function_input; pAct function_input; pErr function_input; okPos function_output; lista function_input; p function_input; pointrit function_output; distPR function_output; position function_input; p1 function_input; p2 function_input; phi function_input; theta function_input; rotation function_output; psi function_input; p1 function_input; p2 function_input; valDist function_output; pRef function_input; pAct function_input; pErr function_input; okPos function_output; p function_input; o function_input; pt function_output; d function_input; distPR function_output; position function_input; p1 function_input; p2 function_input; rit function_output; current_state output size=[1, 8] =[0 0 0 0 0 0 0 0]; pos_ref output =pointP; orient_ref output size=[1 3] =[0 0 deg2rad(angle)]; pos input; orient input; vel input; FLS_front input; FLS_down input; time input; vel_ref output =[0 0 0 0 0 0]; orientA parameter; velPos parameter; velSub parameter; velSurf parameter; velTran parameter; wpEmerg local size=[200 3] =zeros(200,3); altitude parameter; averageDepth parameter; nTran parameter; nWPTran parameter; nWPTurn parameter; pointP parameter; trWP parameter; turnWP parameter; velRid parameter; idxEmerg local =1; missionEnd local =0; endDiv parameter; turnRef parameter; velRidSub parameter; errOrDiv parameter; errOrSurf parameter; errOrTrans parameter; errOrWPTrans parameter; errPosDiv parameter; errPosSurf parameter; errPosTrans parameter; errPosWPTrans parameter; errVelDiv parameter; errVelSurf parameter; inactivity local =1; errOrPos parameter; errPosPos parameter; vEmergTran parameter; offset parameter; sizeEmerg local size=[1,2] =[0 0]; distEmerg parameter; pointA parameter; wpTR local =1; wpTU local =1; page local =1; maxRatio parameter; minDist parameter; minGap parameter; profs local size=[1 20] =zeros(1,20); semix parameter; semiy parameter double; semiz parameter; theta_f parameter; distObsVeh local size=1 =0; distDown local size=1 =0; distFront local size=1 =0; nedAxis local size=[1,3] =zeros(1,3); nedFLS local; pointApp local size=[1,2] =zeros(1,2); pointProf local size=[1 1] =0; distObs local size=1 =0; safeMargin parameter; orDes parameter; orBene local; velNull local; errSphere parameter; ptx local =[0 0 0]; lineSpaceBetweenTransects parameter; ptSup local size=[1 3] =zeros(1,3); orDesRit parameter; orDispari parameter; orPari parameter; fromFirstPos local; wall local =0; rot parameter; errPosTransLast parameter; error local; offsetLast parameter; punto local size=[1 3]; oDeg local; points local size=[20,2] =[]; cruiseSpeed parameter
  function M = currentSwingWaypoints(puntoDes,puntoCorr,dist):
    | function M = currentSwingWaypoints(puntoDes,puntoCorr,dist)
    | %Generazione di waypoint aggiuntivi supponendo di conoscere il punto finale
    | % desiderato sul transetto
    | %
    | %   -puntoDes: punto desiderato sulla traiettoria rettilinea; 1x3 [m m m]
    | %   -puntoCorr: punto stimato di posizione corrente; 1x3 [m m m]
    | %   -dist: distanza tra waypoint; [m]
    | 
    | %     %lunghezza segmento
    | %     lunghezza= sqrt((puntoCorr(1) - puntoDes(1))^2 +(puntoCorr(2)-puntoDes(2))^2);% + (puntoCorr(3) - puntoDes(3))^2); 
    | %     
    | %     p = floor(lunghezza/dist); %numero waypoint
    | 
    |     distN = puntoCorr(1) - puntoDes(1); %distanza su N tra punto iniziale e finale
    |     distE = puntoCorr(2) - puntoDes(2); %distanza su E tra punto iniziale e finale
    | %     distD = puntoCorr(3) - puntoDes(3); %distanza su D tra punto iniziale e finale
    | 
    |     p = floor(abs(distE)/dist);
    |     
    |     deltaE = distE/p; %distanza tra waypoints su East
    |     deltaN = distN/p; %distanza tra waypoints su North
    | %     deltaD = distD/p; %distanza tra waypoints su Down
    |    
    |     matrix = zeros(p-1,3);
    |    
    |     for i = 1:p-1 %possiamo fermarci a p-1 perché waypoint su traiettoria già fornito
    |         waypoint = puntoCorr - i * [deltaN deltaE 0];
    |         waypoint(3) = puntoDes(3);%deltaD];
    |         matrix(i,:) = waypoint;%matrix = cat(1, matrix, waypoint);
    |     end
    |     %matrix = cat(2, matrix, puntoDes);
    |     M = matrix;   
    |    
    | end
  function okVel = checkVel(vRef,vAct,vErr):
    | function okVel = checkVel(vRef,vAct,vErr)
    | %Funzione che controlla che il posizionamento sull'angolo dell'area interessata
    | % sia effettivamente avvenuto, per segnalare l'inizio della fase di
    | % immersione
    | %   -vRef: velocità desiderata; 1x6 [m/s m/s m/s rad/s rad/s rad/s]
    | %   -vAct: velocità corrente; 1x3 [m/s m/s m/s rad/s rad/s rad/s]
    | %   -vErr: errore accettabile in velocità; 1x3 [m/s m/s m/s rad/s rad/s rad/s]
    | 
    |     okVel = all(abs(vRef - vAct) <= vErr); %check su velocità
    | end
  function okOr = checkOr(oRef,oAct,oErr):
    | function okOr = checkOr(oRef,oAct,oErr)
    | %Funzione che controlla che il posizionamento sull'angolo dell'area interessata
    | % sia effettivamente avvenuto, per segnalare l'inizio della fase di
    | % immersione
    | %   -oRef: orientazione desiderata; 1x3 [° ° °]
    | %   -oAct: orientazione corrente, stimata dalla navigazione; 1x3 [° ° °]
    | %   -oErr: errore accettabile in orientamento; 1x3 [° ° °]
    | 
    |     okOr = all(abs(oRef - oAct) <= oErr); %check su orientazione
    | end
  function okPos = checkPos(pRef,pAct,pErr):
    | function okPos = checkPos(pRef,pAct,pErr)
    | %Funzione che controlla che il posizionamento sull'angolo dell'area interessata
    | % sia effettivamente avvenuto, per segnalare l'inizio della fase di
    | % immersione
    | %   -pRef: punto di arrivo desiderato; 1x3 [m m m]
    | %   -pAct: posizione corrente, stimata dalla navigazione; 1x3 [m m m]
    | %   -pErr: errore accettabile in posizione; 1x3 [m m m]
    | 
    |     okPos = all(abs(pRef(1:2) - pAct(1:2))  <= pErr(1:2)); %check su posizione
    | end
  function okPos = checkPos3(pRef,pAct,pErr):
    | function okPos = checkPos3(pRef,pAct,pErr)
    | %Funzione che controlla che il posizionamento sull'angolo dell'area interessata
    | % sia effettivamente avvenuto, per segnalare l'inizio della fase di
    | % immersione
    | %   -pRef: punto di arrivo desiderato; 1x3 [m m m]
    | %   -pAct: posizione corrente, stimata dalla navigazione; 1x3 [m m m]
    | %   -pErr: errore accettabile in posizione; 1x3 [m m m]
    | 
    |     okPos = all(abs(pRef - pAct)  <= pErr); %check su posizione
    | end
  function pointrit = addP(lista,p):
    | function pointrit = addP(lista,p)
    |     if ~all(size(lista))
    |         app = [];
    |         pointrit = cat(1,app,p);
    |     else
    |         pointrit = cat(1,lista,p);
    |     end
    | end
  function distPR = retta(position,p1,p2):
    | function distPR = retta(position,p1,p2)
    | %Funzione che ritorna la distanza tra un punto e una retta costruita a
    | % partire da due suoi punti 
    |     m = p2-p1;
    |     coeff=m(2)/m(1);
    |     distPR = abs(position(2)-(coeff*(position(1)-p1(1))+p1(2)))/sqrt(1+coeff^2);
    |     %y-y1 = m*(x-x1) -> y = m*(x-x1)+y1
    | end
  function rotation = fix2LocalNED(phi, theta, psi):
    | function rotation = fix2LocalNED(phi, theta, psi)
    | %Matrice di rotazione generica per una rotazione RPY, da sdr fisso a sdr
    | %ruotato
    | %   -phi: angolo su asse x
    | %   -theta: angolo su asse y
    | %   -psi: angolo su asse z
    | 
    |     phirad = deg2rad(phi);
    |     cr = cos(phirad);
    |     sr = sin(phirad);
    | 
    |     thetarad = deg2rad(theta);
    |     cp = cos(thetarad);
    |     sp = sin(thetarad);
    | 
    |     psirad = deg2rad(psi);
    |     cy = cos(psirad);
    |     sy = sin(psirad);
    | 
    |     rotx = [[1 0 0];
    |             [0 cr sr];
    |             [0 -sr cr]];
    | 
    |     roty = [[cp 0 -sp];
    |             [0 1 0];
    |             [sp 0 cp]];
    | 
    |     rotz = [[cy sy 0];
    |             [-sy cy 0];
    |             [0 0 1]];
    | 
    |     rotation = rotx*roty*rotz;
    | 
    | end
  function valDist = distance(p1,p2):
    | function valDist = distance(p1,p2)
    |  %p1,p2 considerati di due dimensioni
    |     valDist = sqrt((p1(1)-p2(1))^2 + (p1(2)-p2(2))^2);
    | end
  function okPos = checkPos(pRef,pAct,pErr):
    | function okPos = checkPos(pRef,pAct,pErr)
    | %Funzione che controlla che il posizionamento sull'angolo dell'area interessata
    | % sia effettivamente avvenuto, per segnalare l'inizio della fase di
    | % immersione
    | %   -pRef: punto di arrivo desiderato; 1x3 [m m m]
    | %   -pAct: posizione corrente, stimata dalla navigazione; 1x3 [m m m]
    | %   -pErr: errore accettabile in posizione; 1x3 [m m m]
    | 
    |     okPos = all(abs(pRef(1:2) - pAct(1:2))  <= pErr(1:2)); %check su posizione
    | end
  function pt = calcPoint(p,o,d):
    | function pt = calcPoint(p,o,d)
    |     nedDist = fix2LocalNED(o(1),o(2),o(3))'*[d; 0; 0];
    |     pt = [p(1) p(2)] + [nedDist(1) nedDist(2)];
    |     
    | end
  function distPR = retta(position,p1,p2):
    | function distPR = retta(position,p1,p2)
    | %Funzione che ritorna la distanza tra un punto e una retta costruita a
    | % partire da due suoi punti 
    |     m = p2-p1;
    |     coeff=m(2)/m(1);
    |     distPR = abs(position(2)-(coeff*(position(1)-p1(1))+p1(2)))/sqrt(1+coeff^2);
    |     %y-y1 = m*(x-x1) -> y = m*(x-x1)+y1
    | end

== matlab function TeamA_PAsqualo1/Mission Supervisor2/Trasf. in NED ==
  data: posArg input; pos output; areaOfInterestCorner parameter
function pos = LLD2NED(posArg,areaOfInterestCorner)
    coder.extrinsic('evalin','wgs84Ellipsoid','geodetic2ned');
    pos = zeros(1,3);
    pos1 = 0;
    pos2 = 0;
    pos3 = 0;
    [pos1, pos2, pos3] = geodetic2ned(posArg(1), posArg(2), posArg(3),areaOfInterestCorner(1), areaOfInterestCorner(2), 0,wgs84Ellipsoid);
    pos = [pos1, pos2, posArg(3)];
end

== matlab function TeamA_PAsqualo1/Mission Supervisor2/Trasf. in NED1 ==
  data: posArg input; pos output; areaOfInterestCorner parameter
function pos = NED2LLD(posArg,areaOfInterestCorner)
    coder.extrinsic('evalin','wgs84Ellipsoid','ned2geodetic');
    pos = zeros(1,3);
    pos1 = 0;
    pos2 = 0;
    pos3 = 0;
    [pos1, pos2, pos3] = ned2geodetic(posArg(1), posArg(2), posArg(3),areaOfInterestCorner(1), areaOfInterestCorner(2), 0,wgs84Ellipsoid);
    pos = [pos1, pos2, posArg(3)];%-posArg(3)];
end

== matlab function TeamA_PAsqualo1/geo2ned1 ==
  data: geo input; ned output size=[3 1]; ned_origin parameter
function ned = geo2ned(geo, ned_origin)
coder.extrinsic('evalin', 'wgs84Ellipsoid', 'geodetic2ned');

[x, y, ~] = geodetic2ned(geo(1), geo(2), -geo(3),ned_origin(1), ned_origin(2), ned_origin(3), wgs84Ellipsoid);

ned = zeros(3,1);
ned = [x;y;geo(3)];
end

== matlab function TeamA_PAsqualo1/Controllo Sbaglia segno su Depth ==
  data: u input size=[3 1]; y output
function y = depth2alt(u)

y = zeros(3,1);

y = u;

y(3) = -u(3);

end
